simulink model "SMC_DTC"  (R2023b)
settings: Solver=ode23tb  StartTime=0.0  StopTime=0.4  MaxStep=0.00001  RelTol=1e-4
libraries: spsDCVoltageSourceLib x1, spsGroundLib x1, simulink x1, spsThreePhaseVIMeasurementLib x1, spsUniversalBridgeLib x1, sps_lib x1
settings Model: Creator=rainy  LastModifiedBy=rainy
settings SolverCC: ZeroCrossAlgorithm=Adaptive
settings DebuggingCC: IgnoredZcDiagnostic=none

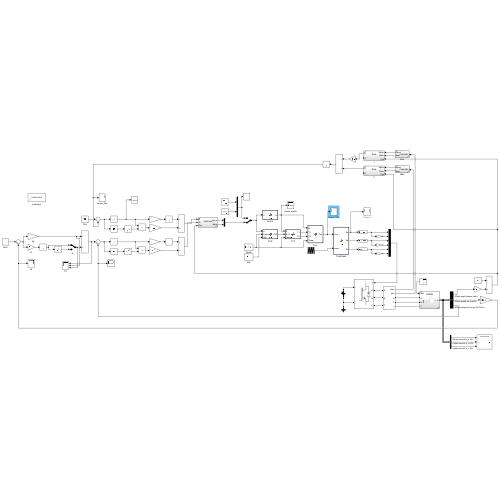
[thumbnail: Simulink's stored preview of the top-level diagram]
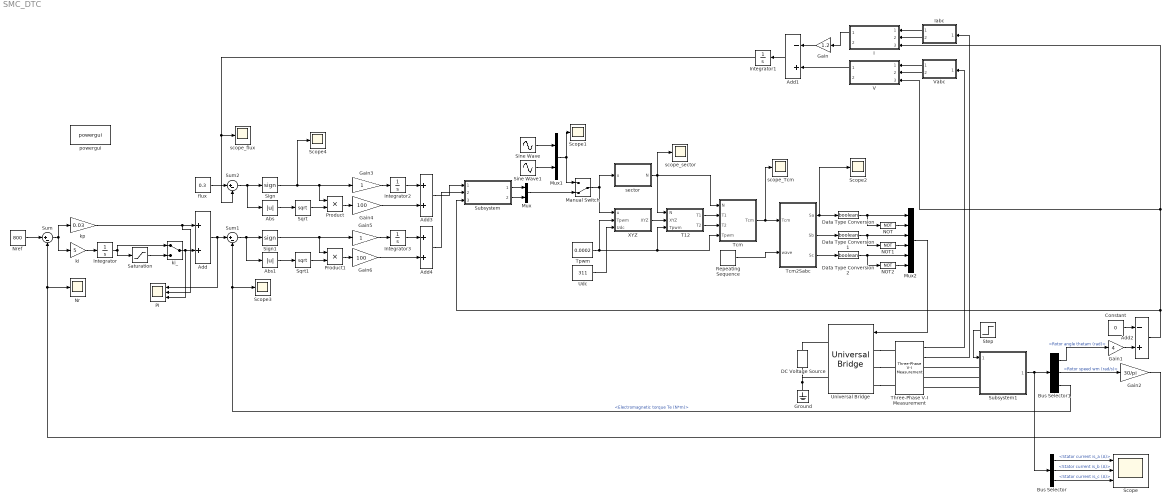
== system SMC_DTC ==
  Abs : Abs  SaturateOnIntegerOverflow=off
  Abs1 : Abs  SaturateOnIntegerOverflow=off
  Add : Sum
  Add1 : Sum  Inputs=-+
  Add2 : Sum  Inputs=-+
  Add3 : Sum
  Add4 : Sum
  Bus Selector : BusSelector  OutputSignals=Stator current is_a (A),Stator current is_b (A),Stator current is_c (A)
  Bus Selector1 : BusSelector  OutputSignals=Rotor angle thetam (rad),Rotor speed wm (rad/s),Electromagnetic torque Te (N*m)
  Constant : Constant  Value=0
  DC Voltage Source : spsDCVoltageSourceLib/DC Voltage Source  Amplitude=311  Measurements=Voltage
  Data Type Conversion : DataTypeConversion  OutDataTypeStr=boolean  SaturateOnIntegerOverflow=off  RndMeth=Floor
  Data Type Conversion1 : DataTypeConversion  OutDataTypeStr=boolean  SaturateOnIntegerOverflow=off  RndMeth=Floor
  Data Type Conversion2 : DataTypeConversion  OutDataTypeStr=boolean  SaturateOnIntegerOverflow=off  RndMeth=Floor
  Gain : Gain  Gain=1.2
  Gain1 : Gain  Gain=4
  Gain2 : Gain  Gain=30/pi
  Gain3 : Gain
  Gain4 : Gain  Gain=100
  Gain5 : Gain
  Gain6 : Gain  Gain=100
  Ground : spsGroundLib/Ground  LConnTagsString=a
  I : Subsystem  ReferencedSubsystem=Park
  Iabc : Subsystem  ReferencedSubsystem=Clark
  Integrator{,1..3} (4 alike) : Integrator
  Manual Switch : ManualSwitch  CurrentSetting=0
  Mux : Mux  Inputs=2
  Mux1 : Mux  Inputs=2
  Mux2 : Mux  Inputs=6
  NOT : Logic  Operator=NOT  IconShape=distinctive  AllPortsSameDT=off  OutDataTypeStr=boolean
  NOT1 : Logic  Operator=NOT  IconShape=distinctive  AllPortsSameDT=off  OutDataTypeStr=boolean
  NOT2 : Logic  Operator=NOT  IconShape=distinctive  AllPortsSameDT=off  OutDataTypeStr=boolean
  Nr : Scope
  Nref : Constant  Value=800
  PI : Scope  NumInputPorts=3
  Product : Product
  Product1 : Product
  Repeating Sequence : simulink/Sources/Repeating Sequence  rep_seq_t=[0 0.0001 0.0002]  rep_seq_y=[0 0.0001 0]
  Saturation : Saturate  UpperLimit=10  LowerLimit=-10
  Scope : Scope  NumInputPorts=3
  Scope{1..4} (4 alike) : Scope
  Sign : Signum
  Sign1 : Signum
  Sine Wave : Sin  Amplitude=200  Frequency=50*pi  SampleTime=0
  Sine Wave1 : Sin  Amplitude=200  Frequency=50*pi  Phase=pi/2  SampleTime=0
  Sqrt : Sqrt
  Sqrt1 : Sqrt
  Step : Step  Time=0.2  After=2  SampleTime=0
  Subsystem : Subsystem  ReferencedSubsystem=AntiPark
  Subsystem1 : Subsystem  ReferencedSubsystem=PMSM
  Sum : Sum  Inputs=|+-
  Sum1 : Sum  Inputs=|+-
  Sum2 : Sum  Inputs=|+-
  T12 : MATLAB Function  TreatAsAtomicUnit=on
  Tcm : MATLAB Function  TreatAsAtomicUnit=on
  Tcm2Sabc : MATLAB Function  TreatAsAtomicUnit=on
  Three-Phase V-I Measurement : spsThreePhaseVIMeasurementLib/Three-Phase V-I Measurement  VoltageMeasurement=phase-to-ground  SetLabelV=off  LabelV=Vabc  Vpu=off  VpuLL=off  CurrentMeasurement=yes  SetLabelI=off  LabelI=Iabc  Ipu=off  Pbase=100e6  Vbase=500e3  OutputType=Complex  PhasorSimulation=off  PSBequivalent=0
  Tpwm : Constant  Value=0.0002
  Udc : Constant  Value=311
  Universal Bridge : spsUniversalBridgeLib/Universal Bridge  Arms=3  SnubberResistance=1e5  SnubberCapacitance=inf  Device=IGBT / Diodes  Ron=1e-3  Lon=0  ForwardVoltages="[  0  0  ]"  ForwardVoltage=0  GTOparameters=[ 10e-6 , 20e-6 ]  IGBTparameters=[ 1e-6 , 2e-6 ]  Measurements=None  Measurements_2=None  converterType=Rectifier
  V : Subsystem  ReferencedSubsystem=Park
  Vabc : Subsystem  ReferencedSubsystem=Clark
  XYZ : MATLAB Function  TreatAsAtomicUnit=on
  flux : Constant  Value=0.3
  ki : Gain  Gain=5
  ki_ : ManualSwitch
  kp : Gain  Gain=0.03
  powergui : sps_lib/powergui  Priority=1  SimulationMode=Continuous  SampleTime=50e-6  frequency=60  Iterations=50  frequencyindice=0  Pbase=100e6  ErrMax=1e-4  UnitsV=kV  UnitsW=MW  buscounter=0  FunctionMessages=off  echomessages=off  EnableUseOfTLC=off  CurrentSourceSwitches=off  DisableSnubberDevices=off  DisableRonSwitches=off  DisableVfSwitches=off  DisplayEquations=off  AutomaticDiscreteSolvers=off  SolverType=Tustin/Backward Euler (TBE)  Interpol=off  ExternalGateDelay=off  methode=off  Ts=100  x0status=blocks  SPID=on  SwTol=0  HookPort=off  NonlinearTolerance=1e-4  nMaxIteration=100  ContinueOnMaxIteration=off  RestoreLinks=warning  ResistiveCurrentMeasurement=off  Frange=[0:2:500]  Ylog=off  Xlog=on  ShowGrid=off  save=off  variable=ZData  structure=0  ZoomFFT=off  StartTime=0.0  cycles=1  DisplayStyle=1  fundamental=60  FreqAxis=off  MaxFrequency=1000  frequencyindicesteady=1  RmsSteady=1  display=off
  scope_Tcm : Scope
  scope_flux : Scope
  scope_sector : Scope
  sector : MATLAB Function  TreatAsAtomicUnit=on
  wires:
  Step/1 -> Subsystem1/1
  Subsystem1/1 -> Bus Selector1/1, Bus Selector/1
  Bus Selector/2 -> Scope/2  "<Stator current is_b (A)>"
  Bus Selector/3 -> Scope/3  "<Stator current is_c (A)>"
  Bus Selector/1 -> Scope/1  "<Stator current is_a (A)>"
  Bus Selector1/2 -> Gain2/1  "<Rotor speed wm (rad/s)>"
  Bus Selector1/3 -> Sum1/2, Scope3/1  "<Electromagnetic torque Te (N*m)>"
  ki_/1 -> PI/3, Add/2
  Saturation/1 -> ki_/2
  Gain2/1 -> Sum/2, Nr/1
  kp/1 -> PI/2, Add/1
  Integrator/1 -> ki_/1, Saturation/1
  ki/1 -> Integrator/1
  Add/1 -> Sum1/1, PI/1
  Sum/1 -> ki/1, kp/1
  Nref/1 -> Sum/1
  Add1/1 -> Integrator1/1
  Three-Phase V-I Measurement/2 -> Iabc/1
  Gain/1 -> Add1/1
  Three-Phase V-I Measurement/1 -> Vabc/1
  Iabc/1 -> I/1
  Iabc/2 -> I/2
  Add2/1 -> V/3, I/3, Subsystem/3
  I/1 -> Gain/1
  Vabc/1 -> V/1
  Vabc/2 -> V/2
  V/1 -> Add1/2
  flux/1 -> Sum2/1
  Integrator1/1 -> Sum2/2, scope_flux/1
  Gain1/1 -> Add2/2
  Constant/1 -> Add2/1
  Bus Selector1/1 -> Gain1/1  "<Rotor angle thetam (rad)>"
  Tpwm/1 -> Tcm/4(Tpwm), T12/3(Tpwm), XYZ/2(Tpwm)
  Udc/1 -> XYZ/3(Udc)
  XYZ/1(XYZ) -> T12/2(XYZ)
  sector/1(N) -> scope_sector/1, Tcm/1(N), T12/1(N)
  T12/1(T1) -> Tcm/2(T1)
  T12/2(T2) -> Tcm/3(T2)
  Tcm/1(Tcm) -> scope_Tcm/1, Tcm2Sabc/1(Tcm)
  Repeating Sequence/1 -> Tcm2Sabc/2(wave)
  NOT/1 -> Mux2/2
  Tcm2Sabc/3(Sc) -> Data Type Conversion2/1
  Data Type Conversion1/1 -> NOT1/1, Mux2/3
  Data Type Conversion2/1 -> NOT2/1, Mux2/5
  Tcm2Sabc/2(Sb) -> Data Type Conversion1/1
  Tcm2Sabc/1(Sa) -> Scope2/1, Data Type Conversion/1
  NOT1/1 -> Mux2/4
  Mux2/1 -> Universal Bridge/1
  Data Type Conversion/1 -> NOT/1, Mux2/1
  NOT2/1 -> Mux2/6
  Subsystem/1 -> Mux/1
  Subsystem/2 -> Mux/2
  Manual Switch/1 -> XYZ/1(u), sector/1(u)
  Mux/1 -> Manual Switch/2
  Mux1/1 -> Scope1/1, Manual Switch/1
  Sine Wave/1 -> Mux1/1
  Sine Wave1/1 -> Mux1/2
  Product/1 -> Gain4/1
  Sqrt/1 -> Product/2
  Abs/1 -> Sqrt/1
  Sign/1 -> Scope4/1, Product/1, Gain3/1
  Gain3/1 -> Integrator2/1
  Integrator2/1 -> Add3/1
  Gain4/1 -> Add3/2
  Sign1/1 -> Product1/1, Gain5/1
  Sqrt1/1 -> Product1/2
  Abs1/1 -> Sqrt1/1
  Gain6/1 -> Add4/2
  Product1/1 -> Gain6/1
  Integrator3/1 -> Add4/1
  Gain5/1 -> Integrator3/1
  Sum1/1 -> Abs1/1, Sign1/1
  Sum2/1 -> Abs/1, Sign/1
  Add3/1 -> Subsystem/1
  Add4/1 -> Subsystem/2
  connections:
  Ground/LConn1 -- Universal Bridge/RConn2 -- DC Voltage Source/LConn1
  Universal Bridge/LConn3 -- Three-Phase V-I Measurement/LConn3
  Subsystem1/LConn3 -- Three-Phase V-I Measurement/RConn3
  Subsystem1/LConn1 -- Three-Phase V-I Measurement/RConn1
  Universal Bridge/LConn2 -- Three-Phase V-I Measurement/LConn2
  Subsystem1/LConn2 -- Three-Phase V-I Measurement/RConn2
  Universal Bridge/LConn1 -- Three-Phase V-I Measurement/LConn1
  DC Voltage Source/RConn1 -- Universal Bridge/RConn1

== matlab function SMC_DTC/XYZ ==
  data: u input; XYZ output; Tpwm input; Udc input
function XYZ = fcn(u, Tpwm, Udc)

XYZ = zeros([1 3]);
XYZ(1) = Tpwm/Udc * sqrt(3)*u(2);
XYZ(2) = Tpwm/Udc * (3/2*u(1) + sqrt(3)/2*u(2));
XYZ(3) = Tpwm/Udc * (-3/2*u(1) + sqrt(3)/2*u(2));

== matlab function SMC_DTC/sector ==
  data: u input; N output
function N = fcn(u)

if(u(1) == 0)
    i = 4;
else
    % 将\psi_{\aplha}和\psi_{\beta}分解为三相
    a1 = u(2);
    b1 = u(2)*(-0.5) + sqrt(3)/2*u(1);
    c1 = u(2)*(-0.5) - sqrt(3)/2*u(1);

    if(a1 > 0)
        a = 1;
    else
        a = 0;
    end
    
    if(b1 > 0)
        b = 1;
    else
        b = 0;
    end
    
    if(c1 > 0)
        c = 1;
    else
        c = 0;
    end

    % i = 4*a+2*b+c;
    i = 4*c+2*b+a;
end

% Sector_table=[4 6 5 2 3 1];
% 
% N = Sector_table(i);
N = i;

== matlab function SMC_DTC/T12 ==
  data: N input; XYZ input; T1 output; Tpwm input; T2 output
function [T1, T2] = fcn(N, XYZ, Tpwm)

X = XYZ(1);
Y = XYZ(2);
Z = XYZ(3);

switch (N)
    case 1
        T1 = Z; T2 = Y;
    case 2
        T1 = Y; T2 = -X;
    case 3
        T1 = -Z; T2 = X;
    case 4
        T1 = -X; T2 = Z;
    case 5
        T1 = X; T2 = -Y;
    otherwise
        T1 = -Y; T2 = -Z;
end

if T1 + T2 > Tpwm
    T1 = T1/(T1 + T2)*Tpwm;
    T2 = T2/(T1 + T2)*Tpwm;
end

== matlab function SMC_DTC/Tcm ==
  data: N input; T1 input; T2 input; Tcm output; Tpwm input
function Tcm = fcn(N, T1, T2, Tpwm)

Tcm = zeros([1 3]);

Ta = (Tpwm - T1 - T2)/4;
Tb = Ta + T1/2;
Tc = Tb + T2/2;

switch(N)
    case 1
        Tcm(1) = Tb;
        Tcm(2) = Ta;
        Tcm(3) = Tc;
    case 2
        Tcm(1) = Ta;
        Tcm(2) = Tc;
        Tcm(3) = Tb;
    case 3
        Tcm(1) = Ta;
        Tcm(2) = Tb;
        Tcm(3) = Tc;
    case 4
        Tcm(1) = Tc;
        Tcm(2) = Tb;
        Tcm(3) = Ta;
    case 5
        Tcm(1) = Tc;
        Tcm(2) = Ta;
        Tcm(3) = Tb;
    otherwise
        Tcm(1) = Tb;
        Tcm(2) = Tc;
        Tcm(3) = Ta;
end

== matlab function SMC_DTC/Tcm2Sabc ==
  data: Tcm input; wave input; Sa output; Sb output; Sc output
function [Sa, Sb, Sc]= fcn(Tcm, wave)

if(wave - Tcm(1) > 0)
    Sa = 1;
else
    Sa = 0;
end

if(wave - Tcm(2) > 0)
    Sb = 1;
else
    Sb = 0;
end

if(wave - Tcm(3) > 0)
    Sc = 1;
else
    Sc = 0;
end
